simulink model "ten_pendulum_sl"  (R2022b)
settings: Solver=ode15s  StartTime=0.0  StopTime=runtime  MaxStep=1e-2  RelTol=1e-3  EnableMultiTasking=on
model workspace (MATLAB code in the model file):
  | m1 = 2;
  | m2 = 3;
  | L1 = 1.2;
  | L2 = 1.6;
  | g = 9.81;
  | theta1_0 = 22.5;
  | theta2_0 = -22.5;
values from neighbouring files (symbols this model uses):
  M1 = Simulink.Parameter(100.0)    [variables.m]
  M10 = Simulink.Parameter(100.0)    [variables.m]
  M2 = Simulink.Parameter(100.0)    [variables.m]
  M3 = Simulink.Parameter(100.0)    [variables.m]
  M4 = Simulink.Parameter(100.0)    [variables.m]
  M5 = Simulink.Parameter(100.0)    [variables.m]
  M6 = Simulink.Parameter(100.0)    [variables.m]
  M7 = Simulink.Parameter(100.0)    [variables.m]
  M8 = Simulink.Parameter(100.0)    [variables.m]
  M9 = Simulink.Parameter(100.0)    [variables.m]
undefined symbols (not defined in the file or in its folder): X, Y, Z
libraries: sm_lib x53, nesl_utility x31
(part 2 of 2)

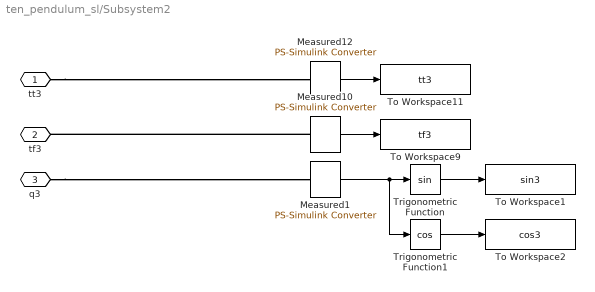
== system ten_pendulum_sl/Subsystem2 ==
  Measured1 : nesl_utility/PS-Simulink Converter  PhysicalDomain=network_engine_domain  SubClassName=ps_output  LeftPortType=input  RightPortType=output  PseudoPeriodic=off  Frequencies=[]  VectorFormat=1-D array  Unit=1  AffineConversion=off
  Measured10 : nesl_utility/PS-Simulink Converter  PhysicalDomain=network_engine_domain  SubClassName=ps_output  LeftPortType=input  RightPortType=output  PseudoPeriodic=off  Frequencies=[]  VectorFormat=1-D array  Unit=1  AffineConversion=off
  Measured12 : nesl_utility/PS-Simulink Converter  PhysicalDomain=network_engine_domain  SubClassName=ps_output  LeftPortType=input  RightPortType=output  PseudoPeriodic=off  Frequencies=[]  VectorFormat=1-D array  Unit=1  AffineConversion=off
  To Workspace1 : ToWorkspace  VariableName=sin3  SampleTime=sampletime
  To Workspace11 : ToWorkspace  VariableName=tt3  SampleTime=sampletime
  To Workspace2 : ToWorkspace  VariableName=cos3  SampleTime=sampletime
  To Workspace9 : ToWorkspace  VariableName=tf3  SampleTime=sampletime
  Trigonometric Function : Trigonometry
  Trigonometric Function1 : Trigonometry  Operator=cos
  tt3 : PMIOPort  Side=Left
  tf3 : PMIOPort  Port=2  Side=Left
  q3 : PMIOPort  Port=3  Side=Left
  wires:
  Measured10/1 -> To Workspace9/1
  Measured12/1 -> To Workspace11/1
  Trigonometric Function/1 -> To Workspace1/1
  Measured1/1 -> Trigonometric Function1/1, Trigonometric Function/1
  Trigonometric Function1/1 -> To Workspace2/1
  connections:
  Measured10/LConn1 -- tf3/RConn1
  tt3/RConn1 -- Measured12/LConn1
  q3/RConn1 -- Measured1/LConn1

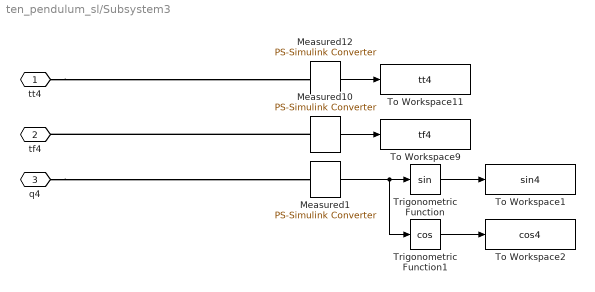
== system ten_pendulum_sl/Subsystem3 ==
  Measured1 : nesl_utility/PS-Simulink Converter  PhysicalDomain=network_engine_domain  SubClassName=ps_output  LeftPortType=input  RightPortType=output  PseudoPeriodic=off  Frequencies=[]  VectorFormat=1-D array  Unit=1  AffineConversion=off
  Measured10 : nesl_utility/PS-Simulink Converter  PhysicalDomain=network_engine_domain  SubClassName=ps_output  LeftPortType=input  RightPortType=output  PseudoPeriodic=off  Frequencies=[]  VectorFormat=1-D array  Unit=1  AffineConversion=off
  Measured12 : nesl_utility/PS-Simulink Converter  PhysicalDomain=network_engine_domain  SubClassName=ps_output  LeftPortType=input  RightPortType=output  PseudoPeriodic=off  Frequencies=[]  VectorFormat=1-D array  Unit=1  AffineConversion=off
  To Workspace1 : ToWorkspace  VariableName=sin4  SampleTime=sampletime
  To Workspace11 : ToWorkspace  VariableName=tt4  SampleTime=sampletime
  To Workspace2 : ToWorkspace  VariableName=cos4  SampleTime=sampletime
  To Workspace9 : ToWorkspace  VariableName=tf4  SampleTime=sampletime
  Trigonometric Function : Trigonometry
  Trigonometric Function1 : Trigonometry  Operator=cos
  tt4 : PMIOPort  Side=Left
  tf4 : PMIOPort  Port=2  Side=Left
  q4 : PMIOPort  Port=3  Side=Left
  wires:
  Measured10/1 -> To Workspace9/1
  Measured12/1 -> To Workspace11/1
  Trigonometric Function/1 -> To Workspace1/1
  Measured1/1 -> Trigonometric Function1/1, Trigonometric Function/1
  Trigonometric Function1/1 -> To Workspace2/1
  connections:
  Measured10/LConn1 -- tf4/RConn1
  tt4/RConn1 -- Measured12/LConn1
  q4/RConn1 -- Measured1/LConn1

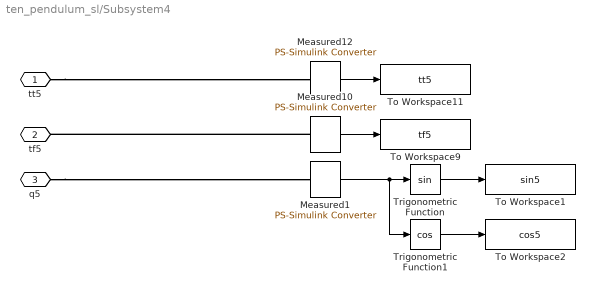
== system ten_pendulum_sl/Subsystem4 ==
  Measured1 : nesl_utility/PS-Simulink Converter  PhysicalDomain=network_engine_domain  SubClassName=ps_output  LeftPortType=input  RightPortType=output  PseudoPeriodic=off  Frequencies=[]  VectorFormat=1-D array  Unit=1  AffineConversion=off
  Measured10 : nesl_utility/PS-Simulink Converter  PhysicalDomain=network_engine_domain  SubClassName=ps_output  LeftPortType=input  RightPortType=output  PseudoPeriodic=off  Frequencies=[]  VectorFormat=1-D array  Unit=1  AffineConversion=off
  Measured12 : nesl_utility/PS-Simulink Converter  PhysicalDomain=network_engine_domain  SubClassName=ps_output  LeftPortType=input  RightPortType=output  PseudoPeriodic=off  Frequencies=[]  VectorFormat=1-D array  Unit=1  AffineConversion=off
  To Workspace1 : ToWorkspace  VariableName=sin5  SampleTime=sampletime
  To Workspace11 : ToWorkspace  VariableName=tt5  SampleTime=sampletime
  To Workspace2 : ToWorkspace  VariableName=cos5  SampleTime=sampletime
  To Workspace9 : ToWorkspace  VariableName=tf5  SampleTime=sampletime
  Trigonometric Function : Trigonometry
  Trigonometric Function1 : Trigonometry  Operator=cos
  tt5 : PMIOPort  Side=Left
  tf5 : PMIOPort  Port=2  Side=Left
  q5 : PMIOPort  Port=3  Side=Left
  wires:
  Measured10/1 -> To Workspace9/1
  Measured12/1 -> To Workspace11/1
  Trigonometric Function/1 -> To Workspace1/1
  Measured1/1 -> Trigonometric Function1/1, Trigonometric Function/1
  Trigonometric Function1/1 -> To Workspace2/1
  connections:
  Measured10/LConn1 -- tf5/RConn1
  tt5/RConn1 -- Measured12/LConn1
  q5/RConn1 -- Measured1/LConn1

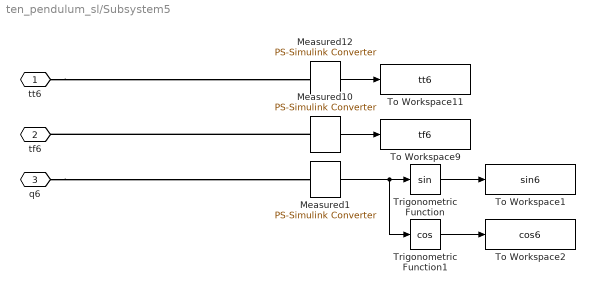
== system ten_pendulum_sl/Subsystem5 ==
  Measured1 : nesl_utility/PS-Simulink Converter  PhysicalDomain=network_engine_domain  SubClassName=ps_output  LeftPortType=input  RightPortType=output  PseudoPeriodic=off  Frequencies=[]  VectorFormat=1-D array  Unit=1  AffineConversion=off
  Measured10 : nesl_utility/PS-Simulink Converter  PhysicalDomain=network_engine_domain  SubClassName=ps_output  LeftPortType=input  RightPortType=output  PseudoPeriodic=off  Frequencies=[]  VectorFormat=1-D array  Unit=1  AffineConversion=off
  Measured12 : nesl_utility/PS-Simulink Converter  PhysicalDomain=network_engine_domain  SubClassName=ps_output  LeftPortType=input  RightPortType=output  PseudoPeriodic=off  Frequencies=[]  VectorFormat=1-D array  Unit=1  AffineConversion=off
  To Workspace1 : ToWorkspace  VariableName=sin6  SampleTime=sampletime
  To Workspace11 : ToWorkspace  VariableName=tt6  SampleTime=sampletime
  To Workspace2 : ToWorkspace  VariableName=cos6  SampleTime=sampletime
  To Workspace9 : ToWorkspace  VariableName=tf6  SampleTime=sampletime
  Trigonometric Function : Trigonometry
  Trigonometric Function1 : Trigonometry  Operator=cos
  tt6 : PMIOPort  Side=Left
  tf6 : PMIOPort  Port=2  Side=Left
  q6 : PMIOPort  Port=3  Side=Left
  wires:
  Measured10/1 -> To Workspace9/1
  Measured12/1 -> To Workspace11/1
  Trigonometric Function/1 -> To Workspace1/1
  Measured1/1 -> Trigonometric Function1/1, Trigonometric Function/1
  Trigonometric Function1/1 -> To Workspace2/1
  connections:
  Measured10/LConn1 -- tf6/RConn1
  tt6/RConn1 -- Measured12/LConn1
  q6/RConn1 -- Measured1/LConn1

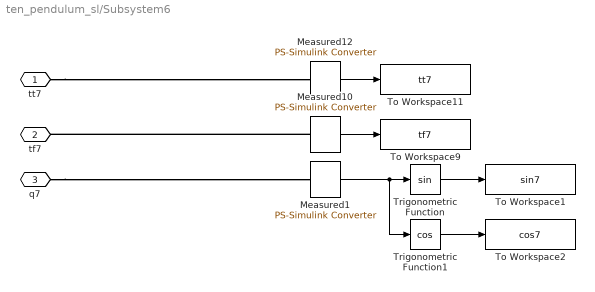
== system ten_pendulum_sl/Subsystem6 ==
  Measured1 : nesl_utility/PS-Simulink Converter  PhysicalDomain=network_engine_domain  SubClassName=ps_output  LeftPortType=input  RightPortType=output  PseudoPeriodic=off  Frequencies=[]  VectorFormat=1-D array  Unit=1  AffineConversion=off
  Measured10 : nesl_utility/PS-Simulink Converter  PhysicalDomain=network_engine_domain  SubClassName=ps_output  LeftPortType=input  RightPortType=output  PseudoPeriodic=off  Frequencies=[]  VectorFormat=1-D array  Unit=1  AffineConversion=off
  Measured12 : nesl_utility/PS-Simulink Converter  PhysicalDomain=network_engine_domain  SubClassName=ps_output  LeftPortType=input  RightPortType=output  PseudoPeriodic=off  Frequencies=[]  VectorFormat=1-D array  Unit=1  AffineConversion=off
  To Workspace1 : ToWorkspace  VariableName=sin7  SampleTime=sampletime
  To Workspace11 : ToWorkspace  VariableName=tt7  SampleTime=sampletime
  To Workspace2 : ToWorkspace  VariableName=cos7  SampleTime=sampletime
  To Workspace9 : ToWorkspace  VariableName=tf7  SampleTime=sampletime
  Trigonometric Function : Trigonometry
  Trigonometric Function1 : Trigonometry  Operator=cos
  tt7 : PMIOPort  Side=Left
  tf7 : PMIOPort  Port=2  Side=Left
  q7 : PMIOPort  Port=3  Side=Left
  wires:
  Measured10/1 -> To Workspace9/1
  Measured12/1 -> To Workspace11/1
  Trigonometric Function/1 -> To Workspace1/1
  Measured1/1 -> Trigonometric Function1/1, Trigonometric Function/1
  Trigonometric Function1/1 -> To Workspace2/1
  connections:
  Measured10/LConn1 -- tf7/RConn1
  tt7/RConn1 -- Measured12/LConn1
  q7/RConn1 -- Measured1/LConn1

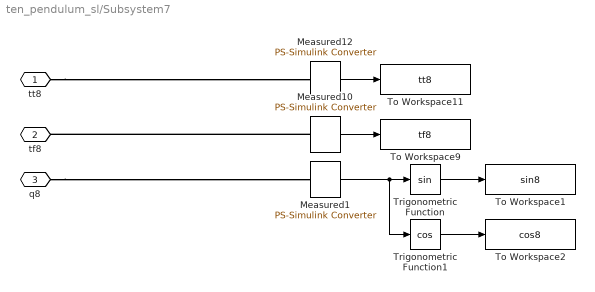
== system ten_pendulum_sl/Subsystem7 ==
  Measured1 : nesl_utility/PS-Simulink Converter  PhysicalDomain=network_engine_domain  SubClassName=ps_output  LeftPortType=input  RightPortType=output  PseudoPeriodic=off  Frequencies=[]  VectorFormat=1-D array  Unit=1  AffineConversion=off
  Measured10 : nesl_utility/PS-Simulink Converter  PhysicalDomain=network_engine_domain  SubClassName=ps_output  LeftPortType=input  RightPortType=output  PseudoPeriodic=off  Frequencies=[]  VectorFormat=1-D array  Unit=1  AffineConversion=off
  Measured12 : nesl_utility/PS-Simulink Converter  PhysicalDomain=network_engine_domain  SubClassName=ps_output  LeftPortType=input  RightPortType=output  PseudoPeriodic=off  Frequencies=[]  VectorFormat=1-D array  Unit=1  AffineConversion=off
  To Workspace1 : ToWorkspace  VariableName=sin8  SampleTime=sampletime
  To Workspace11 : ToWorkspace  VariableName=tt8  SampleTime=sampletime
  To Workspace2 : ToWorkspace  VariableName=cos8  SampleTime=sampletime
  To Workspace9 : ToWorkspace  VariableName=tf8  SampleTime=sampletime
  Trigonometric Function : Trigonometry
  Trigonometric Function1 : Trigonometry  Operator=cos
  tt8 : PMIOPort  Side=Left
  tf8 : PMIOPort  Port=2  Side=Left
  q8 : PMIOPort  Port=3  Side=Left
  wires:
  Measured10/1 -> To Workspace9/1
  Measured12/1 -> To Workspace11/1
  Trigonometric Function/1 -> To Workspace1/1
  Measured1/1 -> Trigonometric Function1/1, Trigonometric Function/1
  Trigonometric Function1/1 -> To Workspace2/1
  connections:
  Measured10/LConn1 -- tf8/RConn1
  tt8/RConn1 -- Measured12/LConn1
  q8/RConn1 -- Measured1/LConn1

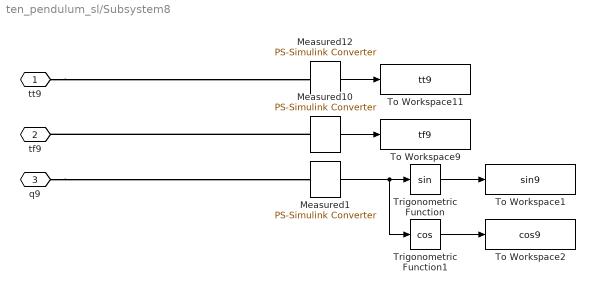
== system ten_pendulum_sl/Subsystem8 ==
  Measured1 : nesl_utility/PS-Simulink Converter  PhysicalDomain=network_engine_domain  SubClassName=ps_output  LeftPortType=input  RightPortType=output  PseudoPeriodic=off  Frequencies=[]  VectorFormat=1-D array  Unit=1  AffineConversion=off
  Measured10 : nesl_utility/PS-Simulink Converter  PhysicalDomain=network_engine_domain  SubClassName=ps_output  LeftPortType=input  RightPortType=output  PseudoPeriodic=off  Frequencies=[]  VectorFormat=1-D array  Unit=1  AffineConversion=off
  Measured12 : nesl_utility/PS-Simulink Converter  PhysicalDomain=network_engine_domain  SubClassName=ps_output  LeftPortType=input  RightPortType=output  PseudoPeriodic=off  Frequencies=[]  VectorFormat=1-D array  Unit=1  AffineConversion=off
  To Workspace1 : ToWorkspace  VariableName=sin9  SampleTime=sampletime
  To Workspace11 : ToWorkspace  VariableName=tt9  SampleTime=sampletime
  To Workspace2 : ToWorkspace  VariableName=cos9  SampleTime=sampletime
  To Workspace9 : ToWorkspace  VariableName=tf9  SampleTime=sampletime
  Trigonometric Function : Trigonometry
  Trigonometric Function1 : Trigonometry  Operator=cos
  tt9 : PMIOPort  Side=Left
  tf9 : PMIOPort  Port=2  Side=Left
  q9 : PMIOPort  Port=3  Side=Left
  wires:
  Measured10/1 -> To Workspace9/1
  Measured12/1 -> To Workspace11/1
  Trigonometric Function/1 -> To Workspace1/1
  Measured1/1 -> Trigonometric Function1/1, Trigonometric Function/1
  Trigonometric Function1/1 -> To Workspace2/1
  connections:
  Measured10/LConn1 -- tf9/RConn1
  tt9/RConn1 -- Measured12/LConn1
  q9/RConn1 -- Measured1/LConn1

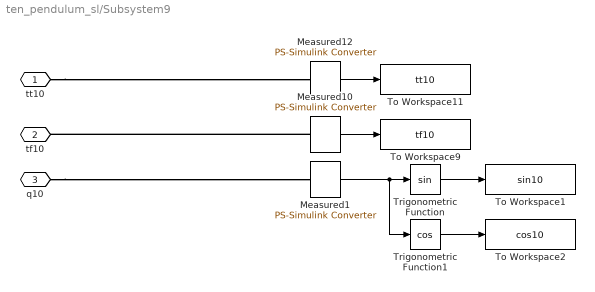
== system ten_pendulum_sl/Subsystem9 ==
  Measured1 : nesl_utility/PS-Simulink Converter  PhysicalDomain=network_engine_domain  SubClassName=ps_output  LeftPortType=input  RightPortType=output  PseudoPeriodic=off  Frequencies=[]  VectorFormat=1-D array  Unit=1  AffineConversion=off
  Measured10 : nesl_utility/PS-Simulink Converter  PhysicalDomain=network_engine_domain  SubClassName=ps_output  LeftPortType=input  RightPortType=output  PseudoPeriodic=off  Frequencies=[]  VectorFormat=1-D array  Unit=1  AffineConversion=off
  Measured12 : nesl_utility/PS-Simulink Converter  PhysicalDomain=network_engine_domain  SubClassName=ps_output  LeftPortType=input  RightPortType=output  PseudoPeriodic=off  Frequencies=[]  VectorFormat=1-D array  Unit=1  AffineConversion=off
  To Workspace1 : ToWorkspace  VariableName=sin10  SampleTime=sampletime
  To Workspace11 : ToWorkspace  VariableName=tt10  SampleTime=sampletime
  To Workspace2 : ToWorkspace  VariableName=cos10  SampleTime=sampletime
  To Workspace9 : ToWorkspace  VariableName=tf10  SampleTime=sampletime
  Trigonometric Function : Trigonometry
  Trigonometric Function1 : Trigonometry  Operator=cos
  tt10 : PMIOPort  Side=Left
  tf10 : PMIOPort  Port=2  Side=Left
  q10 : PMIOPort  Port=3  Side=Left
  wires:
  Measured10/1 -> To Workspace9/1
  Measured12/1 -> To Workspace11/1
  Trigonometric Function/1 -> To Workspace1/1
  Measured1/1 -> Trigonometric Function1/1, Trigonometric Function/1
  Trigonometric Function1/1 -> To Workspace2/1
  connections:
  Measured10/LConn1 -- tf10/RConn1
  tt10/RConn1 -- Measured12/LConn1
  q10/RConn1 -- Measured1/LConn1
